simulink model "QuizRoll"  (R2021b)
settings: Solver=VariableStepAuto  StartTime=0.0  StopTime=5  RelTol=1e-3
values from neighbouring files (symbols this model uses):
  a = 9    [Roll_Optimization_Kp_rootlocus.m]
  b = 33    [Roll_Optimization_Kp_rootlocus.m]
  kp = 0.61    [Roll_Optimization_Kp_rootlocus.m]
  zeta = 0.8    [Roll_Optimization_Kp_rootlocus.m]
settings Model: Creator=oscar  LastModifiedBy=oscar

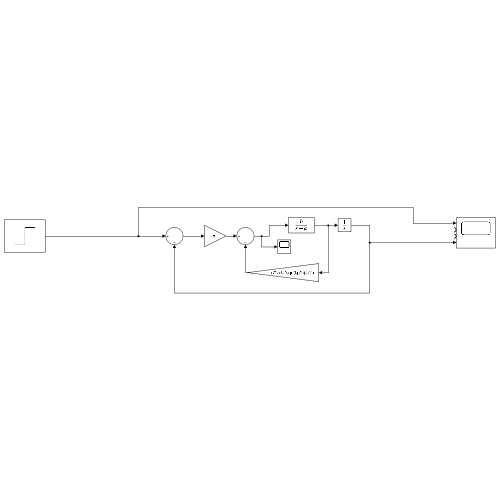
[thumbnail: Simulink's stored preview of the top-level diagram]
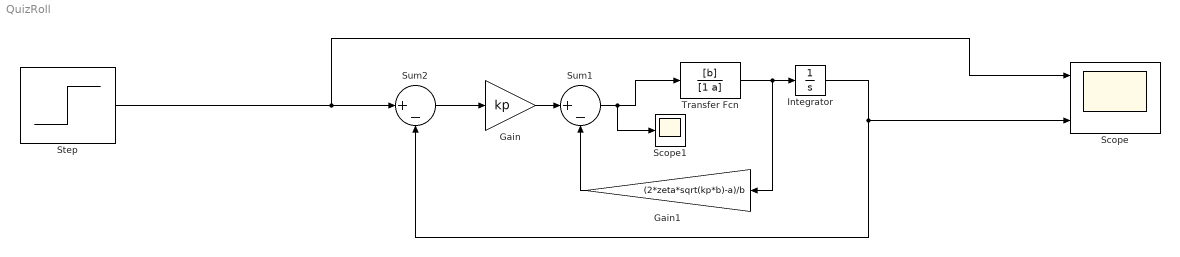
== system QuizRoll ==
  Gain : Gain  Gain=kp  OutMin=0  OutMax=0
  Gain1 : Gain  Gain=(2*zeta*sqrt(kp*b)-a)/b
  Integrator : Integrator
  Scope : Scope  NumInputPorts=4
  Scope1 : Scope
  Step : Step  SampleTime=0
  Sum1 : Sum  Inputs=|+-
  Sum2 : Sum  Inputs=|+-
  Transfer Fcn : TransferFcn  Numerator=[b]  Denominator=[1 a]
  wires:
  Sum2/1 -> Gain/1
  Gain/1 -> Sum1/1
  Sum1/1 -> Scope1/1, Transfer Fcn/1
  Transfer Fcn/1 -> Gain1/1, Integrator/1
  Integrator/1 -> Sum2/2, Scope/4
  Gain1/1 -> Sum1/2
  Step/1 -> Sum2/1, Scope/1
